simulink library "lib_controls"  (Simulink 7.9)
settings: Solver=ode45  SolverMode=SingleTasking  StartTime=0.0  StopTime=10.0  RelTol=1e-3
undefined symbols (not defined in the file or in its folder): amb_tmp, cs_charge_deplete_bool, cs_charge_pwr, cs_charge_trq, cs_clt_tmp, cs_decel_fc_off, cs_decel_regen_threshold, cs_dl_assist_trq_threshold, cs_dl_regen_trq_threshold, cs_electric_decel_spd, cs_electric_launch_spd, cs_electric_launch_spd_hi, cs_electric_launch_spd_lo, cs_eng_min_spd, cs_eng_on_soc, cs_fc_init_state, cs_fc_max_pwr_frac, cs_fc_min_pwr_frac, cs_fc_on, cs_fc_pwr_opt, cs_fc_spd_opt, cs_fuzzy_fuel_mode, cs_hi_soc, cs_hi_trq_frac, cs_lo_soc, cs_lo_trq_frac, cs_max_gc_spd, cs_max_pwr, cs_max_pwr_fall_rate, cs_max_pwr_rise_rate, cs_mc_assist_max_frac, cs_mc_assist_min_frac, cs_mc_assist_slope, cs_mc_regen_max_frac, cs_mc_regen_min_frac, cs_mc_regen_slope, cs_mean_eff, cs_mean_eff_bool, cs_min_gc_spd, cs_min_off_time, cs_min_pwr, cs_min_trq_frac, cs_mph_avg_time, cs_off_trq_frac, cs_plot_output, cs_pwr, cs_regen_avg_time, cs_scale_factor, cs_shutoff, cs_soc_range, cs_spd, cs_target_soc, cs_trq_to_soc_factor, cvt_locus_pwr, cvt_locus_spd, cyc_mph, enable_sim_stop_distance, enable_sim_stop_max_spd, enable_sim_stop_speed, enable_sim_stop_time ... (+110)
libraries: lib_controls x124, simulink3 x13, simulink x5, lib_etc x1
(part 9 of 17)

== system lib_controls/SubSystem/front and rear brake controller (achievable) ==
  total tractive force req'd (N) : Inport
  tractive force available from  front drivetrain (N) : Inport  Port=2
  axle speed possible (rad/s) : Inport  Port=3
  max front brake force (N) : Inport  Port=4
  max rear brake force (N) : Inport  Port=5
  tractive force available from  rear drivetrain (N) : Inport  Port=6
  Block NOTES : Subsystem
      mask Display: disp('Block\nNOTES')
  Constant : Constant  Value=0
  Constant1 : Constant  Value=0
  MinMax : MinMax  Inputs=2  SaturateOnIntegerOverflow=on  InputSameDT=on
  MinMax1 : MinMax  Inputs=2  SaturateOnIntegerOverflow=on  InputSameDT=on
  MinMax2 : MinMax  Function=max  Inputs=2  SaturateOnIntegerOverflow=on  InputSameDT=on
  Sum1 : Sum  Inputs=+--  SaturateOnIntegerOverflow=on  InputSameDT=on  OutDataTypeStr=Inherit: Same as first input
  Sum2 : Sum  Inputs=+-  SaturateOnIntegerOverflow=on  InputSameDT=on  OutDataTypeStr=Inherit: Same as first input
  Switch: braking force to be split between friction brakes (N) : Switch  SaturateOnIntegerOverflow=on  InputSameDT=on
  braking force supplied by front friction brakes (N) : Subsystem
  "m/s -> mph (mph)" : Gain  Gain=2.237  SaturateOnIntegerOverflow=on  OutDataTypeStr=Inherit: Same as input  ParamDataTypeStr=Inherit: Same as input
  "rad/s -> m/s (m/s)" : Gain  Gain=wh_radius  SaturateOnIntegerOverflow=on  OutDataTypeStr=Inherit: Same as input  ParamDataTypeStr=Inherit: Same as input
  rear braking force req'd (N) : Switch  SaturateOnIntegerOverflow=on  InputSameDT=on
  front-axle braking force (N) : Outport  InitialOutput=0
  rear-axle braking force (N) : Outport  Port=2  InitialOutput=0
  wires:
  max rear brake force (N)/1 -> MinMax2/2
  max front brake force (N)/1 -> braking force supplied by front friction brakes (N)/3(max front brake force (N))
  Constant1/1 -> rear braking force req'd (N)/1, MinMax/1
  MinMax/1 -> rear braking force req'd (N)/3
  Sum2/1 -> MinMax/2
  rear braking force req'd (N)/1 -> MinMax2/1
  MinMax2/1 -> rear-axle braking force (N)/1
  "rad/s -> m/s (m/s)"/1 -> "m/s -> mph (mph)"/1
  axle speed possible (rad/s)/1 -> "rad/s -> m/s (m/s)"/1
  tractive force available from  front drivetrain (N)/1 -> Sum1/2
  total tractive force req'd (N)/1 -> Sum1/1, Switch: braking force to be split between friction brakes (N)/2
  Sum1/1 -> MinMax1/2
  MinMax1/1 -> Switch: braking force to be split between friction brakes (N)/3
  Constant/1 -> Switch: braking force to be split between friction brakes (N)/1, MinMax1/1
  "m/s -> mph (mph)"/1 -> braking force supplied by front friction brakes (N)/2(possible speed (mph))
  Switch: braking force to be split between friction brakes (N)/1 -> braking force supplied by front friction brakes (N)/1(add'l braking force req'd (N)), rear braking force req'd (N)/2, Sum2/1
  braking force supplied by front friction brakes (N)/1(braking force from front-axle friction brakes (N)) -> Sum2/2, front-axle braking force (N)/1
  tractive force available from  rear drivetrain (N)/1 -> Sum1/3

== system lib_controls/SubSystem/shifting ==
  gear number : Inport
  Constant : Constant  Value=gb_shift_delay-1e-6
  Relational Operator : RelationalOperator  Operator=<  InputSameDT=on
  time since last shift : Subsystem
      mask Display: disp('time since\nlast shift')
  out_1 : Outport  InitialOutput=0
  wires:
  Relational Operator/1 -> out_1/1
  gear number/1 -> time since last shift/1(in_1)
  Constant/1 -> Relational Operator/2
  time since last shift/1(out_1) -> Relational Operator/1

== system lib_controls/SubSystem/sim stop subsystem ==
  Block NOTES : Subsystem
      mask Display: disp('Block\nNOTES')
  Clock : Clock
  Logical Operator : Logic
  Product{,1..3} (4 alike) : Product  SaturateOnIntegerOverflow=on  RndMeth=Zero  InputSameDT=on  OutDataTypeStr=Inherit: Same as first input
  Relational Operator : RelationalOperator  Operator=>  InputSameDT=on
  Relational Operator1 : RelationalOperator  Operator===  InputSameDT=on
  Stop Simulation : Stop
  Stop Simulation1 : Stop
  Sum : Sum  Inputs=++++  SaturateOnIntegerOverflow=on  InputSameDT=on  OutDataTypeStr=Inherit: Same as first input
  Sum1 : Sum  Inputs=++++  SaturateOnIntegerOverflow=on  InputSameDT=on  OutDataTypeStr=Inherit: Same as first input
  do ex calcs?2 : Constant  Value=enable_stop_fc
  do ex calcs?3 : Constant  Value=enable_sim_stop_distance
  do ex calcs?4 : Constant  Value=enable_sim_stop_speed
  do ex calcs?5 : Constant  Value=enable_sim_stop_time
  do ex calcs?6 : Constant  Value=enable_sim_stop_max_spd
  do ex calcs?7 : Constant  Value=0
  stop sim distance : Subsystem  TreatAsAtomicUnit=on
  stop sim fc : Subsystem  TreatAsAtomicUnit=on
  stop sim max spd : Subsystem  TreatAsAtomicUnit=on
  stop sim speed : Subsystem  TreatAsAtomicUnit=on
  stop sim time : Subsystem  TreatAsAtomicUnit=on
  wires:
  stop sim fc/1(Out1) -> Stop Simulation1/1
  Relational Operator1/1 -> Logical Operator/2
  Relational Operator/1 -> Logical Operator/1
  do ex calcs?7/1 -> Relational Operator/2
  Sum/1 -> Relational Operator/1, Relational Operator1/1
  Sum1/1 -> Relational Operator1/2
  Logical Operator/1 -> Stop Simulation/1
  Product3/1 -> Sum1/4
  Product2/1 -> Sum1/3
  Product1/1 -> Sum1/2
  Product/1 -> Sum1/1
  do ex calcs?6/1 -> Sum/4, Product3/1, stop sim max spd/Enable
  do ex calcs?5/1 -> Sum/3, Product2/1, stop sim time/Enable
  do ex calcs?4/1 -> Sum/2, Product1/1, stop sim speed/Enable
  stop sim speed/1(Out1) -> Product1/2
  stop sim time/1(Out1) -> Product2/2
  stop sim max spd/1(Out1) -> Product3/2
  do ex calcs?3/1 -> Sum/1, Product/1, stop sim distance/Enable
  stop sim distance/1(Out1) -> Product/2
  [mpha] -> stop sim max spd/1(speed)
  Clock/1 -> stop sim time/1(time)
  [mpha] -> stop sim speed/1(speed)
  [distance] -> stop sim distance/1(distance)
  [engine_on] -> stop sim fc/1(engine on?)
  do ex calcs?2/1 -> stop sim fc/Enable

== system lib_controls/SubSystem/traction control ==
  time-average vehicle speed  req'd (m/s) : Inport
  vehicle speed at beginning of time  step (m/s) : Inport  Port=2
  total tractive force req'd (N) : Inport  Port=3
  Block NOTES : Subsystem
      mask Display: disp('Block\nNOTES')
  apply tire traction limit to req'd speed (m/s) : Subsystem
  enforce max.  front axle tractive force  due to slip (N) : Subsystem
  req'd force (N) : Outport  InitialOutput=0
  req'd speed (m/s) : Outport  Port=2  InitialOutput=0
  weight on front axle (N) : Outport  Port=3  InitialOutput=0
  wires:
  time-average vehicle speed  req'd (m/s)/1 -> apply tire traction limit to req'd speed (m/s)/1("requested time-step  average vehicle speed (m/s) ")
  vehicle speed at beginning of time  step (m/s)/1 -> enforce max.  front axle tractive force  due to slip (N)/3(speed at beginning of time step (m/s)), apply tire traction limit to req'd speed (m/s)/2(vehicle speed at beginning of time step (m/s))
  enforce max.  front axle tractive force  due to slip (N)/2(weight on front axle (N)1) -> weight on front axle (N)/1
  enforce max.  front axle tractive force  due to slip (N)/1(slip-limited force (N)) -> req'd force (N)/1
  total tractive force req'd (N)/1 -> enforce max.  front axle tractive force  due to slip (N)/1(tractive force req'd at tire/road interface (N))
  apply tire traction limit to req'd speed (m/s)/1(out_1) -> req'd speed (m/s)/1, enforce max.  front axle tractive force  due to slip (N)/2(requested time-step average vehicle speed (m/s))

== system lib_controls/SubSystem/traction control 2 axle ==
  time-average vehicle speed  req'd (m/s) : Inport
  vehicle speed at beginning of time  step (m/s) : Inport  Port=2
  total tractive force req'd (N) : Inport  Port=3
  Block NOTES : Subsystem
      mask Display: disp('Block\nNOTES')
  apply tire traction limit to req'd speed (m/s) : Subsystem
  enforce max.  front axle tractive force  due to slip (N) : Subsystem
  req'd force (N) : Outport  InitialOutput=0
  req'd speed (m/s) : Outport  Port=2  InitialOutput=0
  weight on front axle (N) : Outport  Port=3  InitialOutput=0
  weight on rear axle (N) : Outport  Port=4  InitialOutput=0
  front/total  traction ratio : Outport  Port=5  InitialOutput=0
  wires:
  apply tire traction limit to req'd speed (m/s)/1(out_1) -> enforce max.  front axle tractive force  due to slip (N)/2(requested time-step average vehicle speed (m/s)), req'd speed (m/s)/1
  total tractive force req'd (N)/1 -> enforce max.  front axle tractive force  due to slip (N)/1(tractive force req'd at tire/road interface (N))
  enforce max.  front axle tractive force  due to slip (N)/1(slip-limited force (N)) -> req'd force (N)/1
  enforce max.  front axle tractive force  due to slip (N)/2(weight on front axle (N)) -> weight on front axle (N)/1
  vehicle speed at beginning of time  step (m/s)/1 -> enforce max.  front axle tractive force  due to slip (N)/3(speed at beginning of time step (m/s)), apply tire traction limit to req'd speed (m/s)/2(vehicle speed at beginning of time step (m/s))
  time-average vehicle speed  req'd (m/s)/1 -> apply tire traction limit to req'd speed (m/s)/1("requested time-step  average vehicle speed (m/s) ")
  enforce max.  front axle tractive force  due to slip (N)/3(weight on rear axle (N)) -> weight on rear axle (N)/1
  enforce max.  front axle tractive force  due to slip (N)/4(front/total traction ratio) -> front/total  traction ratio/1

== system lib_controls/SubSystem/traction control J2452 ==
  time-average vehicle speed  req'd (m/s) : Inport
  vehicle speed at beginning of time  step (m/s) : Inport  Port=2
  total tractive force req'd (N) : Inport  Port=3
  Block NOTES : Subsystem
      mask Display: disp('Block\nNOTES')
  apply tire traction limit to req'd speed (m/s) : Subsystem
  enforce max.  front axle tractive force  due to slip (N) : Subsystem
  req'd force (N) : Outport  InitialOutput=0
  req'd speed (m/s) : Outport  Port=2  InitialOutput=0
  weight on front axle (N) : Outport  Port=3  InitialOutput=0
  wires:
  apply tire traction limit to req'd speed (m/s)/1(out_1) -> enforce max.  front axle tractive force  due to slip (N)/2(requested time-step average vehicle speed (m/s)), req'd speed (m/s)/1
  total tractive force req'd (N)/1 -> enforce max.  front axle tractive force  due to slip (N)/1(tractive force req'd at tire/road interface (N))
  enforce max.  front axle tractive force  due to slip (N)/1(slip-limited force (N)) -> req'd force (N)/1
  enforce max.  front axle tractive force  due to slip (N)/2(weight on front axle (N)1) -> weight on front axle (N)/1
  vehicle speed at beginning of time  step (m/s)/1 -> enforce max.  front axle tractive force  due to slip (N)/3(speed at beginning of time step (m/s)), apply tire traction limit to req'd speed (m/s)/2(vehicle speed at beginning of time step (m/s))
  time-average vehicle speed  req'd (m/s)/1 -> apply tire traction limit to req'd speed (m/s)/1("requested time-step  average vehicle speed (m/s) ")

== system lib_controls/SubSystem/traction control J2452 2 axle ==
  time-average vehicle speed  req'd (m/s) : Inport
  vehicle speed at beginning of time  step (m/s) : Inport  Port=2
  total tractive force req'd (N) : Inport  Port=3
  Block NOTES : Subsystem
      mask Display: disp('Block\nNOTES')
  apply tire traction limit to req'd speed (m/s) : Subsystem
  enforce max.  front axle tractive force  due to slip (N)1 : lib_controls/SubSystem/traction control 2 axle/enforce max.  front axle tractive force  due to slip (N)
      settings: RTWFcnNameOpts=Auto  RTWFileNameOpts=Auto
  req'd force (N) : Outport  InitialOutput=0
  req'd speed (m/s) : Outport  Port=2  InitialOutput=0
  weight on front axle (N) : Outport  Port=3  InitialOutput=0
  weight on rear axle (N) : Outport  Port=4  InitialOutput=0
  front/total  traction ratio : Outport  Port=5  InitialOutput=0
  wires:
  apply tire traction limit to req'd speed (m/s)/1(out_1) -> req'd speed (m/s)/1, enforce max.  front axle tractive force  due to slip (N)1/2
  total tractive force req'd (N)/1 -> enforce max.  front axle tractive force  due to slip (N)1/1
  enforce max.  front axle tractive force  due to slip (N)1/1 -> req'd force (N)/1
  enforce max.  front axle tractive force  due to slip (N)1/2 -> weight on front axle (N)/1
  vehicle speed at beginning of time  step (m/s)/1 -> apply tire traction limit to req'd speed (m/s)/2(vehicle speed at beginning of time step (m/s)), enforce max.  front axle tractive force  due to slip (N)1/3
  time-average vehicle speed  req'd (m/s)/1 -> apply tire traction limit to req'd speed (m/s)/1("requested time-step  average vehicle speed (m/s) ")
  enforce max.  front axle tractive force  due to slip (N)1/3 -> weight on rear axle (N)/1
  enforce max.  front axle tractive force  due to slip (N)1/4 -> front/total  traction ratio/1

== system lib_controls/electric assist control strategy <cs>/chg trq req'd (Nm) ==
  Constant : Constant  Value=cs_charge_trq*fc_trq_scale
  Constant1 : Constant  Value=ess_on
  Goal : Constant  Value=(cs_lo_soc+cs_hi_soc)/2
  Product : Product  SaturateOnIntegerOverflow=on  RndMeth=Zero  InputSameDT=on  OutDataTypeStr=Inherit: Same as first input
  Product1 : Product  Inputs=*/  SaturateOnIntegerOverflow=on  RndMeth=Zero  InputSameDT=on  OutDataTypeStr=Inherit: Same as first input
  Range : Constant  Value=(cs_hi_soc-cs_lo_soc)/2
  Saturation : Saturate  UpperLimit=inf  LowerLimit=-inf
  Sum : Sum  Inputs=-+  SaturateOnIntegerOverflow=on  InputSameDT=on  OutDataTypeStr=Inherit: Same as first input
  Switch : Switch  Threshold=eps  SaturateOnIntegerOverflow=on  InputSameDT=on
  add'l trq req'd (Nm) : Outport
  wires:
  Product/1 -> Saturation/1
  Constant/1 -> Product/1
  Product1/1 -> Product/2
  Sum/1 -> Product1/1
  Range/1 -> Product1/2
  Goal/1 -> Sum/2
  [SOC] -> Sum/1
  Saturation/1 -> Switch/1
  Switch/1 -> add'l trq req'd (Nm)/1
  Constant1/1 -> Switch/2, Switch/3

== system lib_controls/electric assist control strategy <cs>/help ==

== system lib_controls/electric assist control strategy <cs>/minimum trq (Nm) ==
  "trq and spd req'd into trq coupler (N*m, rad/s)" : Inport
  (--) : Constant  Value=cs_lo_soc
  Constant : Constant  Value=0
  Gain : Gain  Gain=cs_min_trq_frac  SaturateOnIntegerOverflow=on  OutDataTypeStr=Inherit: Same as input  ParamDataTypeStr=Inherit: Same as input
  Relational Operator2 : RelationalOperator  Operator=<  InputSameDT=on
  Selector : Selector  InputPortWidth=2  IndexOptions=Index vector (dialog)  Indices=2  OutputSizes=1
  Switch : Switch  Threshold=eps  SaturateOnIntegerOverflow=on  InputSameDT=on
  Terminator : Terminator
  constant threshhold trq (N*m) : Constant  Value=max(fc_max_trq)*0.33
  max_torque lookup : Lookup  InputValues=fc_map_spd  Table=fc_max_trq*fc_trq_scale  SaturateOnIntegerOverflow=on
  minimum trq (N*m) : Outport
  wires:
  [SOC] -> Relational Operator2/1
  (--)/1 -> Relational Operator2/2
  Relational Operator2/1 -> Switch/2
  Switch/1 -> minimum trq (N*m)/1
  Constant/1 -> Switch/3
  constant threshhold trq (N*m)/1 -> Terminator/1
  "trq and spd req'd into trq coupler (N*m, rad/s)"/1 -> Selector/1
  Selector/1 -> max_torque lookup/1
  max_torque lookup/1 -> Gain/1
  Gain/1 -> Switch/1

== system lib_controls/electric assist control strategy bal <cs>/SOC corrected  trq req'd (N*m) ==
  note: This controller produces a modified trq request based on the
      | SOC and the trq request.  The objective is to move the SOC to the
      | mean of the hi and lo set points and to move the trq operation to the
      | mean of the hi and lo trq set points
  "trq and spd req'd into trq coupler (N*m, rad/s)" : Inport
  Abs : Abs  SaturateOnIntegerOverflow=on
  Constant2 : Constant  Value=0
  Constant5 : Constant  Value=-1
  Constant6 : Constant
  Constant7 : Constant  Value=0
  Demux : Demux  Outputs=2
  Gain : Gain  Gain=cs_trq_to_soc_factor  SaturateOnIntegerOverflow=on  OutDataTypeStr=Inherit: Same as input  ParamDataTypeStr=Inherit: Same as input
  Logical Operator1 : Logic  Operator=OR
  Logical Operator2 : Logic  Inputs=3
  Logical Operator3 : Logic
  Logical Operator{4,6,8..9} (4 alike) : Logic  Operator=NOT  Inputs=1
  Logical Operator5 : Logic
  Logical Operator7 : Logic
  Manual  Switch : simulink3/Nonlinear/Manual Switch  sw=1  action=0
  Manual  Switch1 : simulink3/Nonlinear/Manual Switch  sw=1  action=0
  Multiplier4 : Product  Inputs=4  SaturateOnIntegerOverflow=on  RndMeth=Zero  InputSameDT=on  OutDataTypeStr=Inherit: Same as first input
  Relational Operator1 : RelationalOperator  Operator=>  InputSameDT=on
  Relational Operator4 : RelationalOperator  Operator=<  InputSameDT=on
  Relational Operator5 : RelationalOperator  Operator=>  InputSameDT=on
  SOC  Correction  Factor : Subsystem
  Saturation2 : Saturate  UpperLimit=inf  LowerLimit=0
  Sum12 : Sum  SaturateOnIntegerOverflow=on  InputSameDT=on  OutDataTypeStr=Inherit: Same as first input
  Sum13 : Sum  Inputs=-+  SaturateOnIntegerOverflow=on  InputSameDT=on  OutDataTypeStr=Inherit: Same as first input
  Sum14 : Sum  Inputs=2  SaturateOnIntegerOverflow=on  InputSameDT=on  OutDataTypeStr=Inherit: Same as first input
  Sum2 : Sum  Inputs=2  SaturateOnIntegerOverflow=on  InputSameDT=on  OutDataTypeStr=Inherit: Same as first input
  Switch2 : Switch  Threshold=eps  SaturateOnIntegerOverflow=on  InputSameDT=on
  Switch3 : Switch  Threshold=eps  SaturateOnIntegerOverflow=on  InputSameDT=on
  Switch4 : Switch  Threshold=eps  SaturateOnIntegerOverflow=on  InputSameDT=on
  goal SOC1 : Constant  Value=cs_hi_soc
  goal SOC2 : Constant  Value=cs_lo_soc
  goal trq frac : Constant  Value=cs_lo_trq_frac
  goal trq frac1 : Constant  Value=cs_hi_trq_frac
  max trq  and  trq frac : Subsystem
  mean : Gain  Gain=0.5  SaturateOnIntegerOverflow=on  OutDataTypeStr=Inherit: Same as input  ParamDataTypeStr=Inherit: Same as input
  trq  Correction  Factor : Subsystem
  SOC corrected  trq req'd (N*m) : Outport
  wires:
  Gain/1 -> Manual  Switch1/1, Abs/1
  Manual  Switch1/1 -> Sum14/1
  Abs/1 -> Manual  Switch1/2
  Manual  Switch/1 -> Multiplier4/4
  Sum14/1 -> Manual  Switch/1
  goal trq frac/1 -> trq  Correction  Factor/3(low trq), Sum12/2
  max trq  and  trq frac/2(trq frac) -> trq  Correction  Factor/1(trq), Relational Operator5/1, Relational Operator1/2, Sum13/1
  Logical Operator9/1 -> Switch4/2
  Logical Operator1/1 -> Logical Operator9/1
  SOC  Correction  Factor/1(SOC  correction  factor) -> Relational Operator4/2, Manual  Switch/2, Sum14/2
  Constant7/1 -> Switch4/3
  Switch3/1 -> Switch4/1
  Logical Operator7/1 -> Logical Operator1/2
  Logical Operator8/1 -> Logical Operator7/1
  Logical Operator5/1 -> Logical Operator1/1
  Logical Operator6/1 -> Logical Operator5/1
  Logical Operator4/1 -> Logical Operator7/2, Logical Operator3/2
  Constant6/1 -> Switch3/3
  Logical Operator3/1 -> Switch3/2
  Constant5/1 -> Switch3/1
  Constant2/1 -> Relational Operator4/1
  Relational Operator1/1 -> Logical Operator6/1, Logical Operator2/1
  Relational Operator5/1 -> Logical Operator8/1, Logical Operator3/1, Logical Operator2/2
  Logical Operator2/1 -> Switch2/2
  mean/1 -> Relational Operator5/2, Switch2/3
  goal trq frac1/1 -> trq  Correction  Factor/2(high trq), Sum12/1, Relational Operator1/1, Switch2/1
  Sum12/1 -> mean/1
  Switch2/1 -> Sum13/2
  goal SOC2/1 -> SOC  Correction  Factor/3(low soc)
  goal SOC1/1 -> SOC  Correction  Factor/2(high soc)
  [SOC] -> SOC  Correction  Factor/1(SOC)
  Relational Operator4/1 -> Logical Operator5/2, Logical Operator4/1, Logical Operator2/3
  Demux/1 -> max trq  and  trq frac/1(trq req), Sum2/1
  Demux/2 -> max trq  and  trq frac/2(spd req)
  Saturation2/1 -> SOC corrected  trq req'd (N*m)/1
  Sum2/1 -> Saturation2/1
  "trq and spd req'd into trq coupler (N*m, rad/s)"/1 -> Demux/1
  max trq  and  trq frac/1(max trq) -> Multiplier4/1
  Sum13/1 -> Multiplier4/2
  Multiplier4/1 -> Sum2/2
  Switch4/1 -> Multiplier4/3
  trq  Correction  Factor/1(trq  correction  factor) -> Gain/1

== system lib_controls/electric assist control strategy bal <cs>/help ==

== system lib_controls/electric assist control strategy bal <cs>/minimum trq (N*m) ==
  "trq and spd req'd into trq coupler (N*m, rad/s)" : Inport
  Constant : Constant  Value=0
  Gain : Gain  Gain=cs_min_trq_frac  SaturateOnIntegerOverflow=on  OutDataTypeStr=Inherit: Same as input  ParamDataTypeStr=Inherit: Same as input
  Relational Operator2 : RelationalOperator  Operator=<  InputSameDT=on
  Selector : Selector  InputPortWidth=2  IndexOptions=Index vector (dialog)  Indices=2  OutputSizes=1
  Switch : Switch  Threshold=eps  SaturateOnIntegerOverflow=on  InputSameDT=on
  goal SOC : Constant  Value=0.5*(cs_hi_soc+cs_lo_soc)
  max_torque lookup : Lookup  InputValues=fc_map_spd  Table=fc_max_trq*fc_trq_scale  SaturateOnIntegerOverflow=on
  minimum trq (N*m) : Outport
  wires:
  goal SOC/1 -> Relational Operator2/2
  Constant/1 -> Switch/3
  Relational Operator2/1 -> Switch/2
  [SOC] -> Relational Operator2/1
  Gain/1 -> Switch/1
  max_torque lookup/1 -> Gain/1
  Selector/1 -> max_torque lookup/1
  "trq and spd req'd into trq coupler (N*m, rad/s)"/1 -> Selector/1
  Switch/1 -> minimum trq (N*m)/1

== system lib_controls/electric assist control strategy  CVT <cs>/Block NOTES1 ==
  note: Known issues: tm:8/16/00
      | ?? Should inertia estimate be included too??
      | ?? unsure why I must bypass speed calc??

== system lib_controls/electric assist control strategy  CVT <cs>/FC trq and spd ==
  power req'd by FC (W) : Inport
  FC on : Inport  Port=2
  Mode : Inport  Port=3
  Block NOTES : Subsystem
      mask Display: disp('Block\nNOTES')
  Constant : Constant  Value=eps
  Constant5 : Constant  Value=0
  Constant8 : Constant  Value=3
  Mux : Mux  Inputs=2
  Relational Operator1 : RelationalOperator  Operator===  InputSameDT=on
  Saturation3 : Saturate  UpperLimit=max(ptc_fc_mc_iol_pwr_vec)  LowerLimit=min(ptc_fc_mc_iol_pwr_vec)
  Saturation7 : Saturate  UpperLimit=max(ptc_fc_iol_pwr_vec)  LowerLimit=min(ptc_fc_iol_pwr_vec)
  Speed Interp : Subsystem
  Sum : Sum  SaturateOnIntegerOverflow=on  InputSameDT=on  OutDataTypeStr=Inherit: Same as first input
  Sum1 : Sum  SaturateOnIntegerOverflow=on  InputSameDT=on  OutDataTypeStr=Inherit: Same as first input
  Switch1 : Switch  Threshold=eps  SaturateOnIntegerOverflow=on  InputSameDT=on
  To Workspace1 : ToWorkspace  VariableName=cs_pwr_r  SampleTime=-1
  chg pwr req'd (W) : Subsystem
  desired engine trq  mode 3 (Nm) : Product  Inputs=/*  SaturateOnIntegerOverflow=on  RndMeth=Zero  InputSameDT=on  OutDataTypeStr=Inherit: Same as first input
  desired engine trq  mode 4 (Nm) : Lookup  InputValues=ptc_fc_mc_iol_pwr_vec  Table=ptc_fc_mc_iol_trq_vec  SaturateOnIntegerOverflow=on
  mode==3? : Switch  Threshold=eps  SaturateOnIntegerOverflow=on  InputSameDT=on
  mode==4? : Switch  Threshold=3.5  SaturateOnIntegerOverflow=on  InputSameDT=on
  old engine spin up : Subsystem
  "engine torque and speed (Nm), (rad/s)" : Outport  InitialOutput=0
  wires:
  mode==3?/1 -> To Workspace1/1, Saturation7/1, Saturation3/1, Speed Interp/2(pwr req)
  power req'd by FC (W)/1 -> Sum1/2, mode==3?/3
  Sum1/1 -> mode==3?/1
  Relational Operator1/1 -> mode==3?/2
  Constant8/1 -> Relational Operator1/2
  chg pwr req'd (W)/1(add'l pwr req'd (W)) -> Sum1/1
  Mode/1 -> Speed Interp/1(Mode), Relational Operator1/1, mode==4?/2
  Saturation7/1 -> desired engine trq  mode 3 (Nm)/2
  FC on/1 -> Switch1/2, old engine spin up/2(In2)
  Speed Interp/1(input spd) -> Mux/2, old engine spin up/1(In1), Sum/2
  Constant/1 -> Sum/1
  Sum/1 -> desired engine trq  mode 3 (Nm)/1
  Saturation3/1 -> desired engine trq  mode 4 (Nm)/1
  desired engine trq  mode 4 (Nm)/1 -> mode==4?/1
  desired engine trq  mode 3 (Nm)/1 -> mode==4?/3
  Mux/1 -> "engine torque and speed (Nm), (rad/s)"/1
  Switch1/1 -> Mux/1
  mode==4?/1 -> Switch1/1
  Constant5/1 -> Switch1/3

== system lib_controls/electric assist control strategy  CVT <cs>/help ==

== system lib_controls/electric assist control strategy  CVT <cs>/minimum trq (Nm) ==
  "trq and spd req'd into trq coupler (N*m, rad/s)" : Inport
  (--) : Constant  Value=cs_lo_soc
  Constant : Constant  Value=0
  Gain : Gain  Gain=cs_min_trq_frac  SaturateOnIntegerOverflow=on  OutDataTypeStr=Inherit: Same as input  ParamDataTypeStr=Inherit: Same as input
  Relational Operator2 : RelationalOperator  Operator=<  InputSameDT=on
  Selector : Selector  InputPortWidth=2  IndexOptions=Index vector (dialog)  Indices=2  OutputSizes=1
  Switch : Switch  Threshold=eps  SaturateOnIntegerOverflow=on  InputSameDT=on
  Terminator : Terminator
  constant threshhold trq (N*m) : Constant  Value=max(fc_max_trq)*0.33
  max_torque lookup : Lookup  InputValues=fc_map_spd  Table=fc_max_trq*fc_trq_scale  SaturateOnIntegerOverflow=on
  minimum trq (N*m) : Outport
  wires:
  Gain/1 -> Switch/1
  max_torque lookup/1 -> Gain/1
  Selector/1 -> max_torque lookup/1
  "trq and spd req'd into trq coupler (N*m, rad/s)"/1 -> Selector/1
  constant threshhold trq (N*m)/1 -> Terminator/1
  Constant/1 -> Switch/3
  Switch/1 -> minimum trq (N*m)/1
  Relational Operator2/1 -> Switch/2
  (--)/1 -> Relational Operator2/2
  [SOC] -> Relational Operator2/1

== system lib_controls/electric assist control strategy  CVT <cs>/mod pwr req ==
  In1 : Inport
  Sum : Sum  SaturateOnIntegerOverflow=on  InputSameDT=on  OutDataTypeStr=Inherit: Same as first input
  Out1 : Outport
  wires:
  Sum/1 -> Out1/1
  In1/1 -> Sum/1
  [acc_mech_pwr_est] -> Sum/2

== system lib_controls/fuel cell adaptive <cs>/Delta SOC expected from regen ==
  Power req'd by bus (W) : Inport
  Soc : Inport  Port=2
  "  " : Constant  Value=0
  " 2" : Constant  Value=0
  Delta SOC : Sum  Inputs=-+  SaturateOnIntegerOverflow=on  InputSameDT=on  OutDataTypeStr=Inherit: Same as first input
  Logical Operator : Logic
  Memory1 : Memory  X0=ess_init_soc
  "Regen " : Switch  Threshold=eps  SaturateOnIntegerOverflow=on  InputSameDT=on
  Regen flag conditions : Constant  Value=0
  Relational Operator : RelationalOperator  Operator=<=  InputSameDT=on
  Relational Operator1 : RelationalOperator  Operator=<  InputSameDT=on
  Saturation : Saturate  UpperLimit=1  LowerLimit=0
  Subsystem : Subsystem  mask(Running Average){n=cs_regen_avg_time}
      mask prompts: n "Averaging Time (s)"
      mask help: Running Average
      mask Help: Output is the average of the last (Averaging Time) seconds of input.
      mask Display: disp('Running\nAverage')
  Delta SOC regen : Outport
  wires:
  Delta SOC/1 -> Saturation/1
  "Regen "/1 -> Subsystem/1(in_1)
  Subsystem/1(out_1) -> Delta SOC regen/1
  Logical Operator/1 -> "Regen "/2
  Soc/1 -> Delta SOC/2, Memory1/1
  Memory1/1 -> Delta SOC/1
  Saturation/1 -> "Regen "/1
  Power req'd by bus (W)/1 -> Relational Operator/1
  "  "/1 -> "Regen "/3
  Relational Operator/1 -> Logical Operator/2
  Relational Operator1/1 -> Logical Operator/1
  Regen flag conditions/1 -> Relational Operator/2
  " 2"/1 -> Relational Operator1/2
  [ess_pwr_out_a] -> Relational Operator1/1

== system lib_controls/fuel cell adaptive <cs>/SOC regulation factor ==
  In1 : Inport
  1 : Constant
  Goal : Constant  Value=(cs_lo_soc+cs_hi_soc)/2
  Product1 : Product  Inputs=*/  SaturateOnIntegerOverflow=on  RndMeth=Zero  InputSameDT=on  OutDataTypeStr=Inherit: Same as first input
  Range : Constant  Value=(cs_hi_soc-cs_lo_soc)/2
  Saturation : Saturate  UpperLimit=1  LowerLimit=-1
  Sum : Sum  Inputs=-+  SaturateOnIntegerOverflow=on  InputSameDT=on  OutDataTypeStr=Inherit: Same as first input
  Switch : Switch  Threshold=eps  SaturateOnIntegerOverflow=on  InputSameDT=on
  between  0.8 and 1.2 : Fcn  Expr=0.2*u+1
  boolean sustaining/depleting : Constant  Value=cs_charge_deplete_bool
  Out1 : Outport
  wires:
  Sum/1 -> Product1/1
  Range/1 -> Product1/2
  Goal/1 -> Sum/2
  In1/1 -> Sum/1
  Product1/1 -> Saturation/1
  Saturation/1 -> between  0.8 and 1.2/1
  boolean sustaining/depleting/1 -> Switch/2
  1/1 -> Switch/1
  between  0.8 and 1.2/1 -> Switch/3
  Switch/1 -> Out1/1

== system lib_controls/fuel cell control strategy <cs>/FC on ==
  ess max pwr would be insufficient : Inport
  SOC : Inport  Port=2
  FC pwr command : Inport  Port=3
  bus pwr req : Inport  Port=4
  Constant : Constant  Value=cs_hi_soc
  Constant1 : Constant  Value=cs_min_pwr*fc_pwr_scale
  Constant10 : Constant  Value=cs_fc_on
  Constant11 : Constant  Value=0
  Constant2 : Constant  Value=cs_lo_soc
  Constant3 : Constant  Value=0
  Constant4 : Constant
  Constant5 : Constant  Value=cs_min_off_time
  Constant6 : Constant  Value=1.2*cs_min_pwr*fc_pwr_scale
  Constant7 : Constant  Value=fc_on
  Constant8 : Constant  Value=cs_charge_deplete_bool
  Constant9 : Constant
  Gain : Gain  Gain=0.5  SaturateOnIntegerOverflow=on  OutDataTypeStr=Inherit: Same as input  ParamDataTypeStr=Inherit: Same as input
  Logical Operator : Logic  Operator=OR
  Logical Operator{1,3,5..6,8..9} (6 alike) : Logic
  Logical Operator10 : Logic  Operator=NOT
  Logical Operator11 : Logic  Operator=OR
  Logical Operator13 : Logic  Inputs=3
  Logical Operator2 : Logic  Operator=OR  Inputs=3
  Logical Operator4 : Logic  Operator=OR  Inputs=3
  Logical Operator7 : Logic  Operator=NOT  Inputs=1
  Memory : Memory  X0=cs_fc_init_state
  Relational Operator : RelationalOperator  Operator=<=  InputSameDT=on
  Relational Operator1 : RelationalOperator  InputSameDT=on
  Relational Operator2 : RelationalOperator  Operator=<=  InputSameDT=on
  Relational Operator3 : RelationalOperator  InputSameDT=on
  Relational Operator4 : RelationalOperator  InputSameDT=on
  Relational Operator5 : RelationalOperator  Operator=<=  InputSameDT=on
  Relational Operator6 : RelationalOperator  Operator=<  InputSameDT=on
  Relational Operator7 : RelationalOperator  Operator=>  InputSameDT=on
  Relational Operator8 : RelationalOperator  Operator=<  InputSameDT=on
  Subsystem : Subsystem  mask(Running Average){n=5}
      mask prompts: n "Averaging Time (s)"
      mask help: Running Average
      mask Help: Output is the average of the last (Averaging Time) seconds of input.
      mask Display: disp('Running\nAverage')
  Sum : Sum  SaturateOnIntegerOverflow=on  InputSameDT=on  OutDataTypeStr=Inherit: Same as first input
  Sum2 : Sum  Inputs=-+  SaturateOnIntegerOverflow=on  InputSameDT=on  OutDataTypeStr=Inherit: Same as first input
  Switch : Switch  Threshold=eps  SaturateOnIntegerOverflow=on  InputSameDT=on
  dt : Subsystem
  just shut  down : Subsystem
  no-lag Reset Integrator : Subsystem  mask(No-lag Reset Integrator){initval=0}
      mask prompts: initval "Initial Value"
      mask help: No-lag Reset Integrator
      mask Help: Integrates first input using Euler technique.\nAt the time step that input 2 <> zero,\noutput is reset to input 3.
      mask Display: disp('1/s\nw/ reset\nno lag')
  FC on : Outport
  wires:
  Relational Operator6/1 -> Logical Operator8/2
  Constant9/1 -> Relational Operator6/2
  dt/1(out_1) -> Relational Operator6/1
  Logical Operator8/1 -> Logical Operator4/3
  Constant8/1 -> Logical Operator8/1, Logical Operator7/1
  Switch/1 -> Logical Operator4/1
  Logical Operator1/1 -> Logical Operator6/1, Switch/1
  Logical Operator6/1 -> Switch/3
  Logical Operator7/1 -> Switch/2
  Gain/1 -> Relational Operator5/2
  Sum/1 -> Gain/1
  Constant/1 -> Sum/2, Relational Operator/2
  Constant2/1 -> Sum/1, Relational Operator2/2
  Memory/1 -> just shut  down/1(state), Logical Operator2/1
  Constant5/1 -> Relational Operator3/2
  Relational Operator3/1 -> Logical Operator3/1
  no-lag Reset Integrator/1(out_1) -> Relational Operator3/1
  just shut  down/1(trigger) -> no-lag Reset Integrator/2(in_2)
  Constant3/1 -> no-lag Reset Integrator/3(in_3)
  Constant4/1 -> no-lag Reset Integrator/1(in_1)
  Constant6/1 -> Relational Operator4/2
  Relational Operator4/1 -> Logical Operator3/2
  Subsystem/1(out_1) -> Relational Operator4/1
  Logical Operator3/1 -> Logical Operator2/2
  Logical Operator2/1 -> Logical Operator1/1
  SOC/1 -> Relational Operator5/1, Relational Operator/1, Relational Operator2/1
  Relational Operator1/1 -> Logical Operator/2
  FC pwr command/1 -> Relational Operator1/1, Subsystem/1(in_1)
  ess max pwr would be insufficient/1 -> Logical Operator4/2
  Relational Operator5/1 -> Logical Operator6/2
  Relational Operator2/1 -> Logical Operator2/3
  Relational Operator/1 -> Logical Operator/1
  Constant11/1 -> Relational Operator8/2
  [ess_max_chg_pwr] -> Sum2/1
  bus pwr req/1 -> Relational Operator8/1, Sum2/2
  Sum2/1 -> Relational Operator7/2
  Logical Operator/1 -> Logical Operator1/2
  Logical Operator9/1 -> Logical Operator10/1
  Logical Operator10/1 -> Logical Operator5/2
  Relational Operator7/1 -> Logical Operator9/1
  Relational Operator8/1 -> Logical Operator9/2
  Constant1/1 -> Relational Operator1/2, Relational Operator7/1
  Logical Operator5/1 -> Logical Operator11/1
  Constant10/1 -> Logical Operator11/2
  Logical Operator4/1 -> Logical Operator5/1
  Logical Operator11/1 -> Logical Operator13/2
  [key_on] -> Logical Operator13/1
  Constant7/1 -> Logical Operator13/3
  Logical Operator13/1 -> FC on/1, Memory/1

== system lib_controls/fuel cell control strategy <cs>/FC pwr command, modified by SOC ==
  SOC : Inport
  raw pwr command (W) : Inport  Port=2
  pwr req'd at bus (W) : Inport  Port=3
  Block NOTES : Subsystem
      mask Display: disp('Block\nNOTES')
  Gain : Gain  Gain=cs_charge_pwr  SaturateOnIntegerOverflow=on  OutDataTypeStr=Inherit: Same as input  ParamDataTypeStr=Inherit: Same as input
  Gain1 : Gain  Gain=0.5  SaturateOnIntegerOverflow=on  OutDataTypeStr=Inherit: Same as input  ParamDataTypeStr=Inherit: Same as input
  Gain2 : Gain  Gain=-1  SaturateOnIntegerOverflow=on  OutDataTypeStr=Inherit: Same as input  ParamDataTypeStr=Inherit: Same as input
  Goal SOC : Constant  Value=0.5*(cs_hi_soc+cs_lo_soc)
  MinMax1 : MinMax  Inputs=2  SaturateOnIntegerOverflow=on  InputSameDT=on
  Multiplier : Product  Inputs=*/  SaturateOnIntegerOverflow=on  RndMeth=Zero  InputSameDT=on  OutDataTypeStr=Inherit: Same as first input
  Multiplier1 : Product  SaturateOnIntegerOverflow=on  RndMeth=Zero  InputSameDT=on  OutDataTypeStr=Inherit: Same as first input
  SOC Range : Constant  Value=cs_hi_soc-cs_lo_soc
  Saturation : Saturate  UpperLimit=1  LowerLimit=-1
  Sum : Sum  Inputs=-+  SaturateOnIntegerOverflow=on  InputSameDT=on  OutDataTypeStr=Inherit: Same as first input
  Sum1 : Sum  SaturateOnIntegerOverflow=on  InputSameDT=on  OutDataTypeStr=Inherit: Same as first input
  Sum4 : Sum  Inputs=+-  SaturateOnIntegerOverflow=on  InputSameDT=on  OutDataTypeStr=Inherit: Same as first input
  Switch : Switch  SaturateOnIntegerOverflow=on  InputSameDT=on
  ess state : Constant  Value=ess_on
  pwr command modifed for SOC (W) : Outport
  wires:
  SOC/1 -> Sum/1
  Goal SOC/1 -> Sum/2
  SOC Range/1 -> Gain1/1
  Multiplier/1 -> Saturation/1
  Sum/1 -> Multiplier/1
  Saturation/1 -> Gain/1
  Gain1/1 -> Multiplier/2
  MinMax1/1 -> Switch/1
  Gain/1 -> MinMax1/2, Switch/3
  Gain2/1 -> Switch/2
  raw pwr command (W)/1 -> Sum1/1
  pwr req'd at bus (W)/1 -> Sum4/1, Gain2/1
  [ess_max_chg_pwr] -> Sum4/2
  Sum4/1 -> MinMax1/1
  Sum1/1 -> pwr command modifed for SOC (W)/1
  ess state/1 -> Multiplier1/2
  Switch/1 -> Multiplier1/1
  Multiplier1/1 -> Sum1/2

== system lib_controls/fuel cell control strategy <cs>/FC pwr command, w/ limits enforced ==
  ess max pwr would be insufficient : Inport
  SOC : Inport  Port=2
  FC pwr command : Inport  Port=3
  Constant : Constant  Value=cs_min_pwr*fc_pwr_scale
  Constant1 : Constant  Value=cs_lo_soc
  Constant2 : Constant  Value=cs_max_pwr*fc_pwr_scale
  Logical Operator : Logic  Inputs=3
  Logical Operator1 : Logic  Operator=NOT  Inputs=1
  MinMax : MinMax  Function=max  Inputs=2  SaturateOnIntegerOverflow=on  InputSameDT=on
  MinMax1 : MinMax  Inputs=2  SaturateOnIntegerOverflow=on  InputSameDT=on
  Rate Limiter : RateLimiter  RisingSlewLimit=cs_max_pwr_rise_rate*fc_pwr_scale  FallingSlewLimit=cs_max_pwr_fall_rate*fc_pwr_scale
  Relational Operator : RelationalOperator  InputSameDT=on
  Switch : Switch  Threshold=eps  SaturateOnIntegerOverflow=on  InputSameDT=on
  ess state : Constant  Value=ess_on
  limited FC pwr command (W) : Outport
  wires:
  ess max pwr would be insufficient/1 -> Logical Operator1/1
  Logical Operator1/1 -> Logical Operator/1
  Relational Operator/1 -> Logical Operator/2
  SOC/1 -> Relational Operator/1
  Logical Operator/1 -> Switch/2
  Constant1/1 -> Relational Operator/2
  Rate Limiter/1 -> limited FC pwr command (W)/1
  Switch/1 -> Rate Limiter/1
  MinMax/1 -> Switch/3, MinMax1/2
  MinMax1/1 -> Switch/1
  Constant2/1 -> MinMax1/1
  Constant/1 -> MinMax/2
  FC pwr command/1 -> MinMax/1
  ess state/1 -> Logical Operator/3

== system lib_controls/fuel cell control strategy <cs>/pwr req'd from FC to supply pwr req'd at bus (W) ==
  power req'd by bus (W) : Inport
  Constant2 : Constant  Value=0
  Constant3 : Constant  Value=0
  Relational Operator : RelationalOperator  Operator=>  InputSameDT=on
  Switch : Switch  Threshold=eps  SaturateOnIntegerOverflow=on  InputSameDT=on
  pwr req'd of FC (W) : Outport
  wires:
  power req'd by bus (W)/1 -> Relational Operator/1, Switch/1
  Constant2/1 -> Relational Operator/2
  Constant3/1 -> Switch/3
  Relational Operator/1 -> Switch/2
  Switch/1 -> pwr req'd of FC (W)/1

== system lib_controls/series hybrid control stategy  <cs>/FC on ==
  ess max pwr would be insufficient : Inport
  SOC : Inport  Port=2
  FC pwr command : Inport  Port=3
  bus pwr req : Inport  Port=4
  Constant : Constant  Value=cs_hi_soc
  Constant1 : Constant  Value=cs_min_pwr*fc_spd_scale*fc_trq_scale
  Constant11 : Constant  Value=0
  Constant2 : Constant  Value=cs_lo_soc
  Constant3 : Constant  Value=0
  Constant4 : Constant
  Constant5 : Constant  Value=cs_min_off_time
  Constant6 : Constant  Value=1.2*cs_min_pwr*fc_spd_scale*fc_trq_scale
  Constant7 : Constant  Value=fc_on
  Constant8 : Constant  Value=cs_charge_deplete_bool
  Constant9 : Constant
  Gain : Gain  Gain=0.5  SaturateOnIntegerOverflow=on  OutDataTypeStr=Inherit: Same as input  ParamDataTypeStr=Inherit: Same as input
  Logical Operator : Logic  Operator=OR
  Logical Operator{1,3,6,8..9} (5 alike) : Logic
  Logical Operator10 : Logic  Operator=NOT
  Logical Operator2 : Logic  Operator=OR  Inputs=3
  Logical Operator4 : Logic  Operator=OR  Inputs=3
  Logical Operator5 : Logic  Inputs=4
  Logical Operator7 : Logic  Operator=NOT  Inputs=1
  Memory : Memory  X0=cs_fc_init_state
  Relational Operator : RelationalOperator  Operator=<=  InputSameDT=on
  Relational Operator1 : RelationalOperator  InputSameDT=on
  Relational Operator2 : RelationalOperator  Operator=<=  InputSameDT=on
  Relational Operator3 : RelationalOperator  InputSameDT=on
  Relational Operator4 : RelationalOperator  InputSameDT=on
  Relational Operator5 : RelationalOperator  Operator=<=  InputSameDT=on
  Relational Operator6 : RelationalOperator  Operator=<  InputSameDT=on
  Relational Operator7 : RelationalOperator  Operator=>  InputSameDT=on
  Relational Operator8 : RelationalOperator  Operator=<  InputSameDT=on
  Subsystem : Subsystem  mask(Running Average){n=5}
      mask prompts: n "Averaging Time (s)"
      mask help: Running Average
      mask Help: Output is the average of the last (Averaging Time) seconds of input.
      mask Display: disp('Running\nAverage')
  Sum : Sum  SaturateOnIntegerOverflow=on  InputSameDT=on  OutDataTypeStr=Inherit: Same as first input
  Sum2 : Sum  Inputs=-+  SaturateOnIntegerOverflow=on  InputSameDT=on  OutDataTypeStr=Inherit: Same as first input
  Switch : Switch  Threshold=eps  SaturateOnIntegerOverflow=on  InputSameDT=on
  dt : Subsystem
  just shut  down : Subsystem
  no-lag Reset Integrator : Subsystem  mask(No-lag Reset Integrator){initval=0}
      mask prompts: initval "Initial Value"
      mask help: No-lag Reset Integrator
      mask Help: Integrates first input using Euler technique.\nAt the time step that input 2 <> zero,\noutput is reset to input 3.
      mask Display: disp('1/s\nw/ reset\nno lag')
  FC on : Outport
  wires:
  Constant1/1 -> Relational Operator7/1, Relational Operator1/2
  Relational Operator8/1 -> Logical Operator9/2
  Relational Operator7/1 -> Logical Operator9/1
  Logical Operator10/1 -> Logical Operator5/3
  Constant7/1 -> Logical Operator5/4
  [key_on] -> Logical Operator5/1
  Logical Operator5/1 -> Memory/1, FC on/1
  Logical Operator4/1 -> Logical Operator5/2
  Logical Operator9/1 -> Logical Operator10/1
  Logical Operator/1 -> Logical Operator1/2
  Sum2/1 -> Relational Operator7/2
  bus pwr req/1 -> Sum2/2, Relational Operator8/1
  [ess_max_chg_pwr] -> Sum2/1
  Constant11/1 -> Relational Operator8/2
  Relational Operator/1 -> Logical Operator/1
  Relational Operator2/1 -> Logical Operator2/3
  Relational Operator5/1 -> Logical Operator6/2
  ess max pwr would be insufficient/1 -> Logical Operator4/2
  FC pwr command/1 -> Subsystem/1(in_1), Relational Operator1/1
  Relational Operator1/1 -> Logical Operator/2
  SOC/1 -> Relational Operator2/1, Relational Operator/1, Relational Operator5/1
  Logical Operator2/1 -> Logical Operator1/1
  Logical Operator3/1 -> Logical Operator2/2
  Subsystem/1(out_1) -> Relational Operator4/1
  Relational Operator4/1 -> Logical Operator3/2
  Constant6/1 -> Relational Operator4/2
  Constant4/1 -> no-lag Reset Integrator/1(in_1)
  Constant3/1 -> no-lag Reset Integrator/3(in_3)
  just shut  down/1(trigger) -> no-lag Reset Integrator/2(in_2)
  no-lag Reset Integrator/1(out_1) -> Relational Operator3/1
  Relational Operator3/1 -> Logical Operator3/1
  Constant5/1 -> Relational Operator3/2
  Memory/1 -> Logical Operator2/1, just shut  down/1(state)
  Constant2/1 -> Relational Operator2/2, Sum/1
  Constant/1 -> Relational Operator/2, Sum/2
  Sum/1 -> Gain/1
  Gain/1 -> Relational Operator5/2
  Logical Operator7/1 -> Switch/2
  Logical Operator6/1 -> Switch/3
  Logical Operator1/1 -> Switch/1, Logical Operator6/1
  Switch/1 -> Logical Operator4/1
  Constant8/1 -> Logical Operator7/1, Logical Operator8/1
  Logical Operator8/1 -> Logical Operator4/3
  dt/1(out_1) -> Relational Operator6/1
  Constant9/1 -> Relational Operator6/2
  Relational Operator6/1 -> Logical Operator8/2

== system lib_controls/series hybrid control stategy  <cs>/FC pwr command, modified by SOC ==
  SOC : Inport
  raw pwr command (W) : Inport  Port=2
  pwr req'd at bus (W) : Inport  Port=3
  Block NOTES : Subsystem
      mask Display: disp('Block\nNOTES')
  Gain : Gain  Gain=cs_charge_pwr  SaturateOnIntegerOverflow=on  OutDataTypeStr=Inherit: Same as input  ParamDataTypeStr=Inherit: Same as input
  Gain1 : Gain  Gain=0.5  SaturateOnIntegerOverflow=on  OutDataTypeStr=Inherit: Same as input  ParamDataTypeStr=Inherit: Same as input
  Gain2 : Gain  Gain=-1  SaturateOnIntegerOverflow=on  OutDataTypeStr=Inherit: Same as input  ParamDataTypeStr=Inherit: Same as input
  Goal SOC : Constant  Value=0.5*(cs_hi_soc+cs_lo_soc)
  MinMax1 : MinMax  Inputs=2  SaturateOnIntegerOverflow=on  InputSameDT=on
  Multiplier : Product  Inputs=*/  SaturateOnIntegerOverflow=on  RndMeth=Zero  InputSameDT=on  OutDataTypeStr=Inherit: Same as first input
  Multiplier1 : Product  SaturateOnIntegerOverflow=on  RndMeth=Zero  InputSameDT=on  OutDataTypeStr=Inherit: Same as first input
  SOC Range : Constant  Value=cs_hi_soc-cs_lo_soc
  Saturation : Saturate  UpperLimit=1  LowerLimit=-1
  Sum : Sum  Inputs=-+  SaturateOnIntegerOverflow=on  InputSameDT=on  OutDataTypeStr=Inherit: Same as first input
  Sum1 : Sum  SaturateOnIntegerOverflow=on  InputSameDT=on  OutDataTypeStr=Inherit: Same as first input
  Sum4 : Sum  Inputs=+-  SaturateOnIntegerOverflow=on  InputSameDT=on  OutDataTypeStr=Inherit: Same as first input
  Switch : Switch  SaturateOnIntegerOverflow=on  InputSameDT=on
  ess state : Constant  Value=ess_on
  pwr command modifed for SOC (W) : Outport
  wires:
  Sum4/1 -> MinMax1/1
  [ess_max_chg_pwr] -> Sum4/2
  pwr req'd at bus (W)/1 -> Gain2/1, Sum4/1
  raw pwr command (W)/1 -> Sum1/1
  Gain2/1 -> Switch/2
  Gain/1 -> Switch/3, MinMax1/2
  MinMax1/1 -> Switch/1
  Gain1/1 -> Multiplier/2
  Saturation/1 -> Gain/1
  Sum/1 -> Multiplier/1
  Multiplier/1 -> Saturation/1
  SOC Range/1 -> Gain1/1
  Goal SOC/1 -> Sum/2
  SOC/1 -> Sum/1
  Sum1/1 -> pwr command modifed for SOC (W)/1
  Switch/1 -> Multiplier1/1
  Multiplier1/1 -> Sum1/2
  ess state/1 -> Multiplier1/2

== system lib_controls/series hybrid control stategy  <cs>/FC pwr command, w/ limits enforced ==
  ess max pwr would be insufficient : Inport
  SOC : Inport  Port=2
  FC pwr command : Inport  Port=3
  Constant : Constant  Value=cs_min_pwr*fc_spd_scale*fc_trq_scale
  Constant1 : Constant  Value=cs_lo_soc
  Constant2 : Constant  Value=cs_max_pwr*fc_spd_scale*fc_trq_scale
  Constant3 : Constant  Value=ess_on
  Logical Operator : Logic  Inputs=3
  Logical Operator1 : Logic  Operator=NOT  Inputs=1
  MinMax : MinMax  Function=max  Inputs=2  SaturateOnIntegerOverflow=on  InputSameDT=on
  MinMax1 : MinMax  Inputs=2  SaturateOnIntegerOverflow=on  InputSameDT=on
  Rate Limiter : RateLimiter  RisingSlewLimit=cs_max_pwr_rise_rate*fc_spd_scale*fc_trq_scale  FallingSlewLimit=cs_max_pwr_fall_rate*fc_spd_scale*fc_trq_scale
  Relational Operator : RelationalOperator  InputSameDT=on
  Switch : Switch  Threshold=eps  SaturateOnIntegerOverflow=on  InputSameDT=on
  limited FC pwr command (W) : Outport
  wires:
  ess max pwr would be insufficient/1 -> Logical Operator1/1
  Logical Operator1/1 -> Logical Operator/1
  Relational Operator/1 -> Logical Operator/2
  SOC/1 -> Relational Operator/1
  FC pwr command/1 -> MinMax/1
  MinMax/1 -> Switch/3, MinMax1/2
  Constant/1 -> MinMax/2
  Logical Operator/1 -> Switch/2
  Constant1/1 -> Relational Operator/2
  Rate Limiter/1 -> limited FC pwr command (W)/1
  Switch/1 -> Rate Limiter/1
  MinMax1/1 -> Switch/1
  Constant2/1 -> MinMax1/1
  Constant3/1 -> Logical Operator/3

== system lib_controls/series hybrid control stategy  <cs>/FC trq and spd ==
  FC on : Inport
  power req'd by FC (W) : Inport  Port=2
  Block NOTES : Subsystem
      mask Display: disp('Block\nNOTES')
  Constant : Constant  Value=eps
  Constant5 : Constant  Value=0
  Constant6 : Constant  Value=0
  Constant7 : Constant  Value=eps
  Gain : Gain  Gain=.5  SaturateOnIntegerOverflow=on  OutDataTypeStr=Inherit: Same as input  ParamDataTypeStr=Inherit: Same as input
  Logical Operator : Logic
  Logical Operator1 : Logic  Operator=NOT  Inputs=1
  Memory : Memory
  Mux : Mux  Inputs=2
  Relational Operator : RelationalOperator  Operator=>  InputSameDT=on
  Saturation : Saturate  UpperLimit=max(cs_pwr)  LowerLimit=min(cs_pwr)
  Sum : Sum  SaturateOnIntegerOverflow=on  InputSameDT=on  OutDataTypeStr=Inherit: Same as first input
  Switch1 : Switch  Threshold=eps  SaturateOnIntegerOverflow=on  InputSameDT=on
  Switch2 : Switch  Threshold=eps  SaturateOnIntegerOverflow=on  InputSameDT=on
  Switch3 : Switch  Threshold=eps  SaturateOnIntegerOverflow=on  InputSameDT=on
  desired spd (rad/s) : Lookup  InputValues=cs_pwr  Table=cs_spd  SaturateOnIntegerOverflow=on
  desired trq (Nm) : Product  Inputs=*/  SaturateOnIntegerOverflow=on  RndMeth=Zero  InputSameDT=on  OutDataTypeStr=Inherit: Same as first input
  "engine torque and speed (Nm), (rad/s)" : Outport  InitialOutput=0
  wires:
  Switch3/1 -> Mux/2
  Gain/1 -> Switch3/1
  Switch2/1 -> Switch3/3, Gain/1, Relational Operator/1
  Logical Operator1/1 -> Logical Operator/2
  Relational Operator/1 -> Memory/1, Logical Operator/1
  Memory/1 -> Logical Operator1/1
  Constant7/1 -> Relational Operator/2
  Logical Operator/1 -> Switch3/2
  Switch1/1 -> Mux/1
  Mux/1 -> "engine torque and speed (Nm), (rad/s)"/1
  FC on/1 -> Switch2/2, Switch1/2
  desired spd (rad/s)/1 -> Switch2/1, Sum/2
  Constant6/1 -> Switch2/3
  Constant5/1 -> Switch1/3
  Saturation/1 -> desired trq (Nm)/1, desired spd (rad/s)/1
  power req'd by FC (W)/1 -> Saturation/1
  Constant/1 -> Sum/1
  desired trq (Nm)/1 -> Switch1/1
  Sum/1 -> desired trq (Nm)/2

== system lib_controls/series hybrid control stategy  <cs>/power follower ==
